simulink model "ysw8_9"  (R2014a)
settings: Solver=ode15s  StartTime=0.0  StopTime=0.02  RelTol=1e-3
libraries: powerlib x13
settings Model: Creator=Administrator  LastModifiedBy=Administrator
settings DebuggingCC: UnconnectedInputMsg=none  UnconnectedOutputMsg=none  UnconnectedLineMsg=none

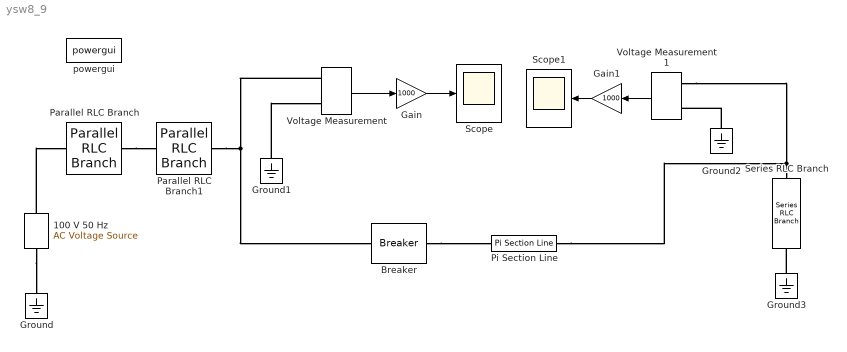
== system ysw8_9 ==
  100 V 50 Hz : powerlib/Electrical Sources/AC Voltage Source  Description=source block  Amplitude=100  Phase=0  Frequency=50  SampleTime=0  Measurements=None
      settings: AttributesFormatString=\n
  Breaker : powerlib/Elements/Breaker  InitialState=0  SwitchingTimes=[1/200]  External=off  BreakerResistance=0.001  SnubberResistance=inf  SnubberCapacitance=0  Measurements=None  MoreParameters=on  NoBreakLoop=off
  Gain : Gain  Gain=1000
  Gain1 : Gain  Gain=1000
  Ground{,1..3} (4 alike) : powerlib/Elements/Ground  LConnTagsString=a
  Parallel RLC Branch : powerlib/Elements/Parallel RLC Branch  LConnTagsString=a  RConnTagsString=__new0  BranchType=R  Resistance=2  Inductance=1e-3  SetiL0=off  InitialCurrent=0  Capacitance=1e-6  Setx0=off  InitialVoltage=0  Measurements=None
  Parallel RLC Branch1 : powerlib/Elements/Parallel RLC Branch  LConnTagsString=a  RConnTagsString=__new0  BranchType=RLC  Resistance=180.1  Inductance=26.525e-3  SetiL0=off  InitialCurrent=0  Capacitance=117.84e-6  Setx0=off  InitialVoltage=0  Measurements=None
  Pi Section Line : powerlib/Elements/Pi Section Line  LConnTagsString=__new0  RConnTagsString=__new0  Frequency=50  Resistance=0.1  Inductance=0.0016  Capacitance=0.0102e-6  Length=300  PiSections=10  Measurements=None
      settings: AttributesFormatString=\n
  Scope : Scope
  Scope1 : Scope
  Series RLC Branch : powerlib/Elements/Series RLC Branch  LConnTagsString=__new0  RConnTagsString=__new0  BranchType=RL  Resistance=1  Inductance=1e-3  SetiL0=off  InitialCurrent=0  Capacitance=1e-6  Setx0=off  InitialVoltage=0  Measurements=None
  Voltage Measurement : powerlib/Measurements/Voltage Measurement  PhasorSimulation=off  OutputType=Complex  PSBequivalent=0
  Voltage Measurement1 : powerlib/Measurements/Voltage Measurement  PhasorSimulation=off  OutputType=Complex  PSBequivalent=0
  powergui : powerlib/powergui  SimulationMode=Continuous  SolverType=Tustin  SampleTime=25e-6  frequency=60  SPID=off  DisableSnubberDevices=off  DisableRonSwitches=off  DisableVfSwitches=off  SwTol=0  Interpol=off  DisplayEquations=off  Ts=0  methode=off  frequencyindice=50  Pbase=100e6  ErrMax=1e-4  Iterations=50  UnitsV=kV  UnitsW=MW  FunctionMessages=off  echomessages=off  HookPort=off  EnableUseOfTLC=off  x0status=blocks  RestoreLinks=warning  ResistiveCurrentMeasurement=off  Frange=[0:2:10000]  Ylog=on  Xlog=off  ShowGrid=on  save=off  variable=ZData  structure=0  ZoomFFT=off  StartTime=0.0  cycles=1  DisplayStyle=1  fundamental=60  FreqAxis=off  MaxFrequency=1000  frequencyindicesteady=1  RmsSteady=1  display=off
  wires:
  Voltage Measurement/1 -> Gain/1
  Gain/1 -> Scope/1
  Voltage Measurement1/1 -> Gain1/1
  Gain1/1 -> Scope1/1
  connections:
  100 V 50 Hz/LConn1 -- Ground/LConn1
  100 V 50 Hz/RConn1 -- Parallel RLC Branch/RConn1
  Ground1/LConn1 -- Voltage Measurement/LConn2
  Voltage Measurement1/LConn1 -- Pi Section Line/RConn1 -- Series RLC Branch/LConn1
  Ground3/LConn1 -- Series RLC Branch/RConn1
  Ground2/LConn1 -- Voltage Measurement1/LConn2
  Breaker/RConn1 -- Pi Section Line/LConn1
  Voltage Measurement/LConn1 -- Parallel RLC Branch1/RConn1 -- Breaker/LConn1
  Parallel RLC Branch/LConn1 -- Parallel RLC Branch1/LConn1
